simulink model "Implicit_TickEvent_Temporal_Logic"  (R2018b)
settings: Solver=FixedStepDiscrete  StartTime=0.0  StopTime=10.0  FixedStep=0.5  RelTol=1e-3
settings Model: Creator=marwan  LastModifiedBy=marwan

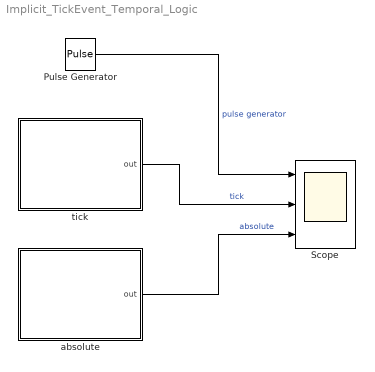
== system Implicit_TickEvent_Temporal_Logic ==
  Pulse Generator : DiscretePulseGenerator  PulseType=Time based  Period=2.5  PulseWidth=60
  Scope : Scope  NumInputPorts=3
  absolute : Stateflow chart  TreatAsAtomicUnit=on
  tick : Stateflow chart  TreatAsAtomicUnit=on
  wires:
  Pulse Generator/1 -> Scope/1  "pulse generator"
  tick/1(out) -> Scope/2  "tick"
  absolute/1(out) -> Scope/3  "absolute"

== stateflow chart Implicit_TickEvent_Temporal_Logic/absolute ==
  state st1
    en:
    out=true;
  state st2
    en:
    out=false;
  (default) -> st1
  st1 -> st2 : [after(1.5,sec)]
  st2 -> st1 : [after(1,sec)]
  data: out output

== stateflow chart Implicit_TickEvent_Temporal_Logic/tick ==
  state st1
    en:
    out=true;
  state st2
    en:
    out=false;
  (default) -> st1
  st1 -> st2 : [after(3,tick)]
  st2 -> st1 : [after(2,tick)]
  data: out output
